simulink model "ModelisationGlobal"  (R2020b)
settings: Solver=VariableStepAuto  StartTime=0.0  StopTime=10.0  RelTol=1e-3
settings Model: Creator=Roxanne Simard  LastModifiedBy=Roxanne Simard

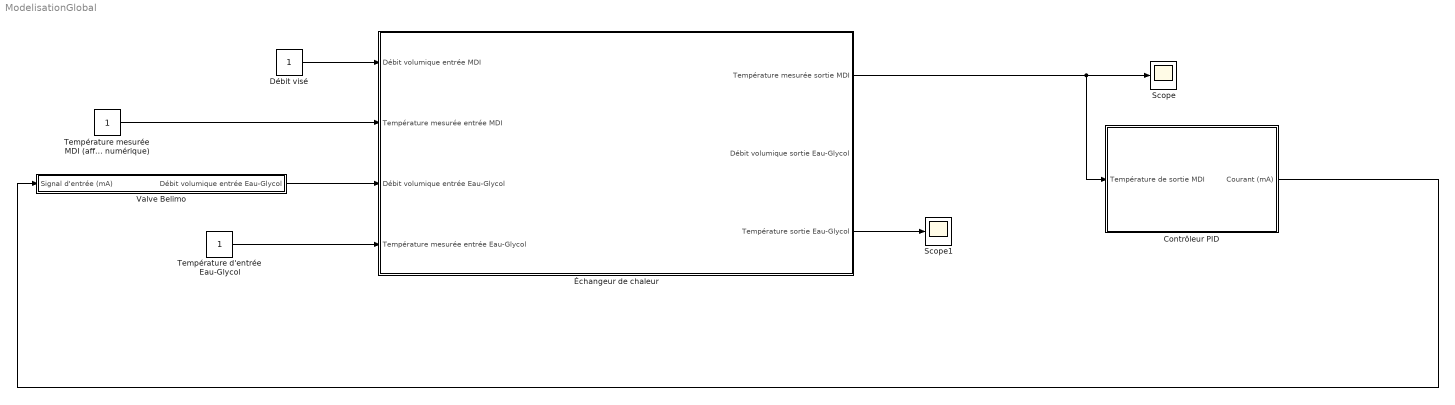
== system ModelisationGlobal ==
  Contrôleur PID : Subsystem
  Débit visé : Constant
  Scope : Scope
  Scope1 : Scope
  Température d'entrée Eau-Glycol : Constant
  Température mesurée MDI (affichage numérique) : Constant
  Valve Belimo : Subsystem
  Échangeur de chaleur : Subsystem
  wires:
  Valve Belimo/1(Débit volumique entrée Eau-Glycol) -> Échangeur de chaleur/3(Débit volumique entrée Eau-Glycol)
  Contrôleur PID/1(Courant (mA)) -> Valve Belimo/1(Signal d'entrée (mA))
  Température mesurée MDI (affichage numérique)/1 -> Échangeur de chaleur/2(Température mesurée entrée MDI)
  Échangeur de chaleur/1(Température mesurée sortie MDI) -> Contrôleur PID/1(Température de sortie MDI), Scope/1
  Température d'entrée Eau-Glycol/1 -> Échangeur de chaleur/4(Température mesurée entrée Eau-Glycol)
  Débit visé/1 -> Échangeur de chaleur/1(Débit volumique entrée MDI)
  Échangeur de chaleur/3(Température sortie Eau-Glycol) -> Scope1/1

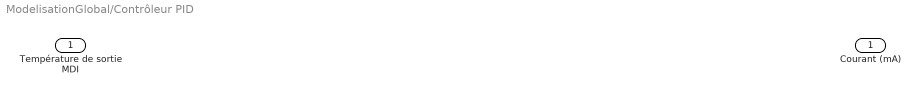
== system ModelisationGlobal/Contrôleur PID ==
  Température de sortie MDI : Inport
  Courant (mA) : Outport

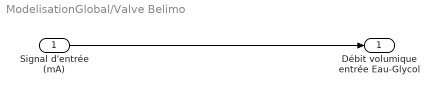
== system ModelisationGlobal/Valve Belimo ==
  Signal d'entrée (mA) : Inport
  Débit volumique entrée Eau-Glycol : Outport
  wires:
  Signal d'entrée (mA)/1 -> Débit volumique entrée Eau-Glycol/1

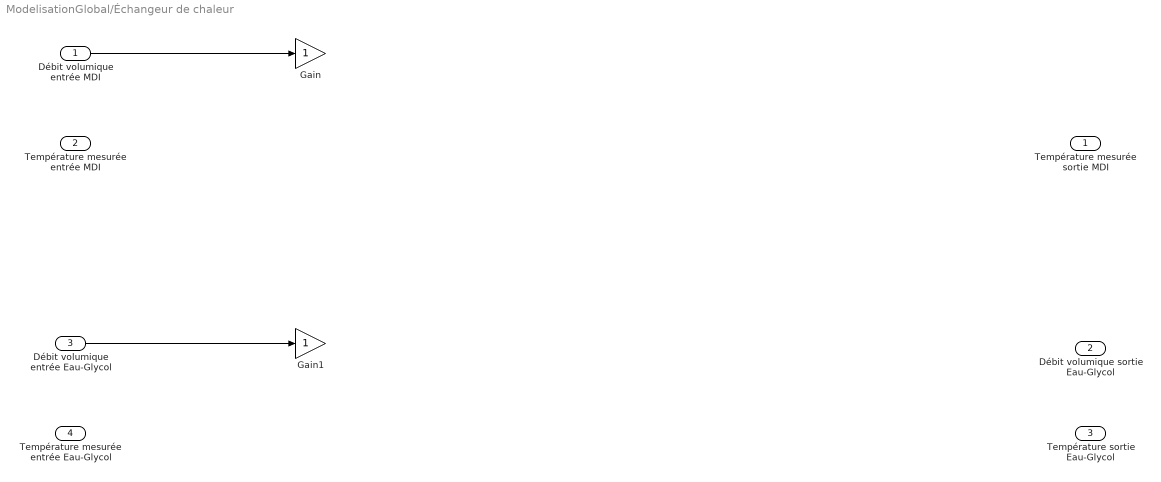
== system ModelisationGlobal/Échangeur de chaleur ==
  Débit volumique entrée MDI : Inport
  Température mesurée entrée MDI : Inport  Port=2
  Débit volumique entrée Eau-Glycol : Inport  Port=3
  Température mesurée entrée Eau-Glycol : Inport  Port=4
  Gain : Gain
  Gain1 : Gain
  Température mesurée sortie MDI : Outport
  Débit volumique sortie Eau-Glycol : Outport  Port=2
  Température sortie Eau-Glycol : Outport  Port=3
  wires:
  Débit volumique entrée MDI/1 -> Gain/1
  Débit volumique entrée Eau-Glycol/1 -> Gain1/1
